simulink model "demorig"  (Simulink 6.1)
settings: Solver=ode45  StartTime=0.0  StopTime=1000  RelTol=1e-3
undefined symbols (not defined in the file): D, slcm
libraries: marine_gnc x3, simulink_extras x2, simulink x1
settings Model: LastModifiedBy=perez
settings DataIOCC: SignalLoggingName=sigsOut
settings OptimizationCC: InlineInvariantSignals=off
settings HardwareCC: TargetUnknown=on
settings CodeAppCC: IgnoreCustomStorageClasses=off
settings GRTTargetCC: ModelReferenceCompliant=off  MatFileLogging=off

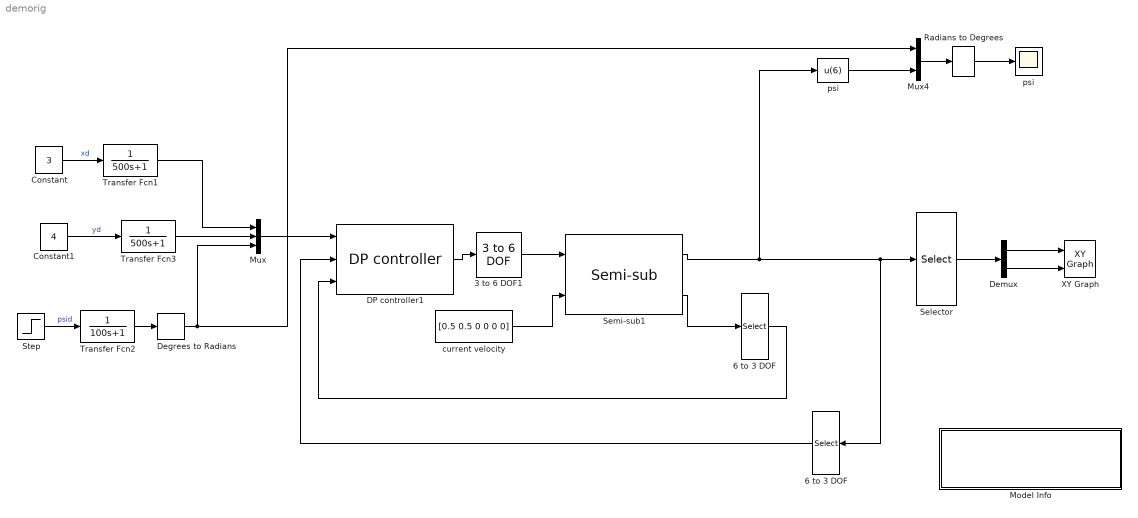
== system demorig ==
  3 to 6 DOF1 : marine_gnc/Models/ Kinetics /Support/3 to 6 DOF
  6 to 3 DOF : Selector  Elements=[1 2 6]  InputPortWidth=6
  "6 to 3 DOF  " : Selector  Orientation=left  Elements=[1 2 6]  InputPortWidth=6
  Constant : Constant  Value=3
  Constant1 : Constant  Value=4
  DP controller1 : marine_gnc/Control/Dynamic  Positioning /DP controller  Kp=diag([0.044e10 0.0069e10 6.9241e10])*0.1*0.1  Kd=diag([0.044e10 0.0069e10 6.9241e10])*2*0.1  Ki=diag([0.044e10 0.0069e10 6.9241e10])*(0.1^3)/10
  Degrees to Radians : simulink_extras/Transformations/Degrees to Radians
  Demux : Demux  Outputs=2
  Model Info : Subsystem  LoadFcn=slcm LoadBlock;  InitFcn=slcm('UpdateAllCMBlocksInThisModelInit')  mask(CMBlock){InitialSaveTempField=, InitialBlockCM=None, BlockCM=None, Frame=on, SaveTempField=, DisplayStringWithTags=|, MaskDisplayString=DP system for a semi-submersible\nexposed for currents. \nAuthor: Thor I. Fossen\n04-Mar-2005 13:00:44, HorizontalTextAlignment=Left, LeftAlignmentValue=0.02, SourceBlockDiagram=demorig, TagMaxNumber=20, CMTag1=, CMTag2=, CMTag3=, CMTag4=, CMTag5=, CMTag6=, CMTag7=, CMTag8=, CMTag9=, CMTag10=, CMTag11=, CMTag12=, CMTag13=, CMTag14=, CMTag15=, CMTag16=, CMTag17=, CMTag18=, CMTag19=, CMTag20=}
      mask DisplayStringWithTags=|
      | DP system for a semi-submersible
      | exposed for currents.
      | %<Creator>Author: Thor I. Fossen
      | %<LastModificationDate>
      mask help: This block allows revision control information to be displayed within the model.
      settings: CopyFcn=slcm CopyBlock;  DeleteFcn=slcm Cancel;  PostSaveFcn=slcm('UpdateAllCMBlocksInThisModel')  NameChangeFcn=slcm Rename;  OpenFcn=slcm
      mask Display: text(str2num(LeftAlignmentValue), 0.5, MaskDisplayString, 'HorizontalAlignment', HorizontalTextAlignment)
  Mux : Mux  Inputs=3
  Mux4 : Mux  Inputs=2
  Radians to Degrees : simulink_extras/Transformations/Radians to Degrees
  Selector : Selector  Elements=[1 2]  InputPortWidth=6
  Semi-sub1 : marine_gnc/Examples/Vessels/Semi-sub  D=D  G=G  MA=MA  MRB=MRB
  Step : Step  Time=30  After=10  SampleTime=0
  Transfer Fcn1 : TransferFcn  Denominator=[500 1]
  Transfer Fcn2 : TransferFcn  Denominator=[100 1]
  Transfer Fcn3 : TransferFcn  Denominator=[500 1]
  XY Graph : simulink/Sinks/XY Graph  xmin=-5  xmax=5  ymin=-5  ymax=5  st=-1
  current velocity : Constant  Value=[0.5 0.5 0 0 0 0]
  psi : Fcn  Expr=u(6)
  "psi  " : Scope
      settings: TimeRange=1000  YMin=-2  YMax=10
  wires:
  Constant/1 -> Transfer Fcn1/1  "xd"
  Step/1 -> Transfer Fcn2/1  "psid"
  Degrees to Radians/1 -> Mux/3, Mux4/1
  Constant1/1 -> Transfer Fcn3/1  "yd"
  Demux/1 -> XY Graph/1
  Demux/2 -> XY Graph/2
  Mux/1 -> DP controller1/1
  Transfer Fcn2/1 -> Degrees to Radians/1
  Semi-sub1/1 -> psi/1, Selector/1, "6 to 3 DOF  "/1
  Radians to Degrees/1 -> "psi  "/1
  Mux4/1 -> Radians to Degrees/1
  DP controller1/1 -> 3 to 6 DOF1/1
  psi/1 -> Mux4/2
  Selector/1 -> Demux/1
  current velocity/1 -> Semi-sub1/2
  3 to 6 DOF1/1 -> Semi-sub1/1
  6 to 3 DOF/1 -> DP controller1/3
  "6 to 3 DOF  "/1 -> DP controller1/2
  Semi-sub1/2 -> 6 to 3 DOF/1
  Transfer Fcn1/1 -> Mux/1
  Transfer Fcn3/1 -> Mux/2

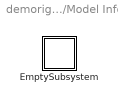
== system demorig/Model Info ==
  EmptySubsystem : Subsystem

== system demorig/Model Info/EmptySubsystem ==
